simulink model "pipline_system"  (R2022b)
settings: Solver=FixedStepAuto  StartTime=0.0  StopTime=2000  FixedStep=Ts  RelTol=1e-5
values from neighbouring files (symbols this model uses):
  Aeq = [A_bar -B_bar ... (first row only)    [run_pipeline_system.m]
  B = -[1;0;0;0]    [myStateTransitionFcn.m]    (also in run_pipeline_system.m = [1;0;0;0])
  B_dem = -[0;0;0;1]    [myStateTransitionFcn.m]    (also in run_pipeline_system.m = [0;0;0;1])
  B_dem_bar = kron(eye(h),B_demd)    [run_pipeline_system.m]
  B_h = -[0 0;1 0;0 1;0 0]    [myStateTransitionFcn.m]    (also in run_pipeline_system.m = [0 0;1 0;0 1;0 0])
  Bh_bar = kron(eye(h),B_hd)    [run_pipeline_system.m]
  c = 330    [myStateTransitionFcn.m]    (also in run_pipeline_system.m)
  h = 10    [run_pipeline_system.m]
  K_control = place(A,B,poles)    [run_pipeline_system.m]
  K_inv = (pi^2)/(64*c^2)*f*D_edge.^5./L_edge    [myStateTransitionFcn.m]    (also in run_pipeline_system.m)
  M = blkdiag(Q_bar, R_bar)    [run_pipeline_system.m]
  n = 4    [run_pipeline_system.m]
  p_eq = [P1;P2;P3;P4]    [run_pipeline_system.m]
  V = (pi/8)*sum(((D_edge.^2).*L_edge),2,'omitnan')    [myStateTransitionFcn.m]    (also in run_pipeline_system.m)
  w_eq = c^2*(sqrt(K_inv.*abs(l*(p_eq.^2).' - (p_eq.^2)*l.')).*sign(l*p_eq.' - p_eq*l.')*l)./V    [run_pipeline_system.m]
undefined symbols (not defined in the file or in its folder): sigbuilder_block
settings Model: Creator=Anubi  LastModifiedBy=digitalstorm
settings ModelReferenceCC: EnableRefExpFcnMdlSchedulingChecks=on

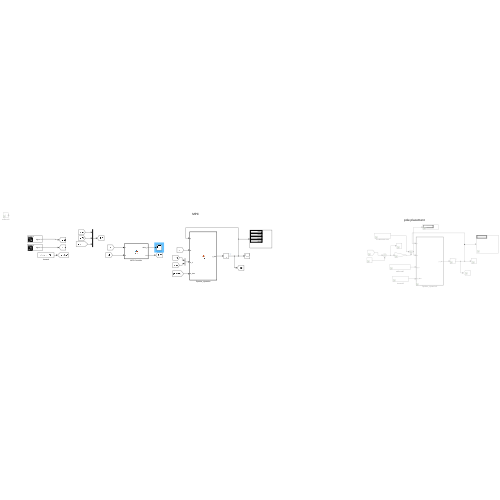
[thumbnail: Simulink's stored preview of the top-level diagram]
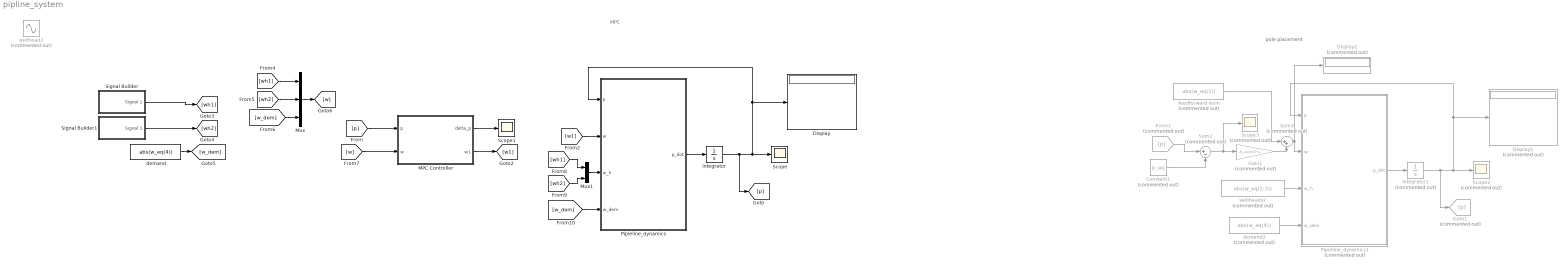
== system pipline_system ==
  note: pole placement
  note: MPC
  Constant1 : Constant  Commented=on  Value=p_eq
  Display : Display
  Display1 : Display  Commented=on
  Display2 : Display  Commented=on
  From1 : From  Commented=on  GotoTag=p
  Gain1 : Gain  Commented=on  Gain=-K_control  Multiplication=Matrix(K*u) (u vector)
  Goto1 : Goto  Commented=on  GotoTag=p
  Integrator : Integrator  InitialCondition=p_eq
  Integrator1 : Integrator  Commented=on  InitialCondition=0.5*p_eq
  MPC Controller : MATLAB Function  TreatAsAtomicUnit=on
  Mux : Mux  Inputs=3
  Mux1 : Mux  Inputs=2
  Pipieline_dynamics : MATLAB Function  TreatAsAtomicUnit=on
  Pipieline_dynamics1 : MATLAB Function  Commented=on  TreatAsAtomicUnit=on
  Scope : Scope
  Scope1 : Scope
  Scope2 : Scope  Commented=on
  Scope3 : Scope  Commented=on
  Signal Builder : Subsystem  Tag=STV Subsys  LoadFcn=sigbuilder_block('load');  StartFcn=sigbuilder_block('start');  StopFcn=sigbuilder_block('stop');  ClipboardFcn=sigbuilder_block('clipboard');  mask(Sigbuilder block){tuvar=[0:10]}
      mask help: Simulink:masks:SigbuilderBlock_MD
      mask init:
      | if ~strcmp(get_param(bdroot(gcbh),'SimulationStatus'),'stopped') tuvar = sigbuilder_block('maskInit'); end
      settings: CopyFcn=sigbuilder_block('copy');  DeleteFcn=sigbuilder_block('delete');  ModelCloseFcn=sigbuilder_block('modelClose');  PreSaveFcn=sigbuilder_block('preSave');  PauseFcn=sigbuilder_block('pause');  ContinueFcn=sigbuilder_block('continue');  NameChangeFcn=sigbuilder_block('namechange');  OpenFcn=sigbuilder_block('open',[428.444 190.222 568.889 387.556 ]);  CloseFcn=sigbuilder_block('close');
      mask Display: plot(0, 0, 100, 100,[2, 2, 32, 32, 2], [68, 8, 8, 68, 68],[32, 2], [38, 38], [32, 19, 2],[53, 60, 44], [32, 17, 17, 2],[16, 16, 31, 31]);txt = getActiveGroup(gcbh);text(2, 100, txt,'verticalAlignment', 'top');
  Signal Builder1 : Subsystem  Tag=STV Subsys  LoadFcn=sigbuilder_block('load');  StartFcn=sigbuilder_block('start');  StopFcn=sigbuilder_block('stop');  ClipboardFcn=sigbuilder_block('clipboard');  mask(Sigbuilder block){tuvar=[0:10]}
      mask help: Simulink:masks:SigbuilderBlock_MD
      mask init:
      | if ~strcmp(get_param(bdroot(gcbh),'SimulationStatus'),'stopped') tuvar = sigbuilder_block('maskInit'); end
      settings: CopyFcn=sigbuilder_block('copy');  DeleteFcn=sigbuilder_block('delete');  ModelCloseFcn=sigbuilder_block('modelClose');  PreSaveFcn=sigbuilder_block('preSave');  PauseFcn=sigbuilder_block('pause');  ContinueFcn=sigbuilder_block('continue');  NameChangeFcn=sigbuilder_block('namechange');  OpenFcn=sigbuilder_block('open',[428.444 190.222 568.889 387.556 ]);  CloseFcn=sigbuilder_block('close');
      mask Display: plot(0, 0, 100, 100,[2, 2, 32, 32, 2], [68, 8, 8, 68, 68],[32, 2], [38, 38], [32, 19, 2],[53, 60, 44], [32, 17, 17, 2],[16, 16, 31, 31]);txt = getActiveGroup(gcbh);text(2, 100, txt,'verticalAlignment', 'top');
  Sum2 : Sum  Commented=on  Inputs=|+-
  Sum3 : Sum  Commented=on  Inputs=|++
  demand : Constant  Value=abs(w_eq(4))
  demand2 : Constant  Commented=on  Value=abs(w_eq(4))
  feedforward term : Constant  Commented=on  Value=abs(w_eq(1))
  wellhead2 : Sin  Commented=on  Amplitude=2.5  Bias=5  Frequency=0.005  SampleTime=0
  wellheads2 : Constant  Commented=on  Value=abs(w_eq(2:3))
  wires:
  Pipieline_dynamics/1(p_dot) -> Integrator/1
  Integrator/1 -> [p], Scope/1, Pipieline_dynamics/1(p), Display/1
  Sum3/1 -> Display2/1, Pipieline_dynamics1/2(w)
  Gain1/1 -> Sum3/2
  feedforward term/1 -> Sum3/1
  demand2/1 -> Pipieline_dynamics1/4(w_dem)
  Sum2/1 -> Scope3/1, Gain1/1
  Integrator1/1 -> Goto1/1, Scope2/1, Pipieline_dynamics1/1(p), Display1/1
  wellheads2/1 -> Pipieline_dynamics1/3(w_h)
  Pipieline_dynamics1/1(p_dot) -> Integrator1/1
  From1/1 -> Sum2/1
  Constant1/1 -> Sum2/2
  [p] -> MPC Controller/1(p)
  MPC Controller/2(w1) -> [w1]
  [w1] -> Pipieline_dynamics/2(w)
  demand/1 -> [w_dem]
  Mux/1 -> [w]
  [w] -> MPC Controller/2(w)
  Mux1/1 -> Pipieline_dynamics/3(w_h)
  [wh1] -> Mux1/1
  [wh2] -> Mux1/2
  [w_dem] -> Pipieline_dynamics/4(w_dem)
  [wh1] -> Mux/1
  [wh2] -> Mux/2
  [w_dem] -> Mux/3
  MPC Controller/1(delta_p) -> Scope1/1
  Signal Builder/1(Signal 1) -> [wh1]
  Signal Builder1/1(Signal 1) -> [wh2]

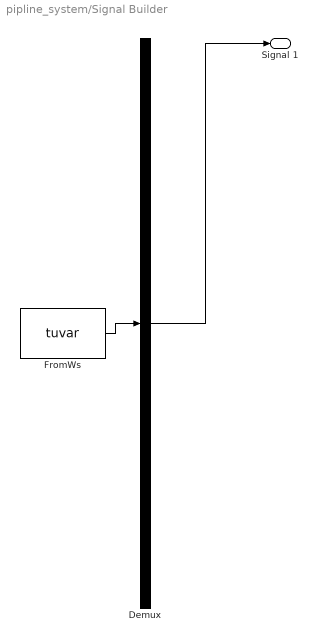
== system pipline_system/Signal Builder ==
  Demux : Demux  Tag=STV Demux  Outputs=1
      settings: DisplayOption=none
  FromWs : FromWorkspace  Tag=STV FromWs  VariableName=tuvar
      SigBuilderData=|
      | common.afterFinalStr = 'Extrapolate'
      | common.sampleTime = 0
      | dataSet.timeRange = [0 2000]
      | dataSet.name = 'Group 1'
      | sbobj.Groups.Name = 'Group 1'
      | sbobj.Groups.Signals.Name = 'Signal 1'
      | sbobj.Groups.Signals.XData = [0 1000 2000]
      | sbobj.Groups.Signals.YData = [5 4.8 5.1]
      | sbobj.Groups.TimeRange = [0 2000]
  Signal 1 : Outport  Tag=STV Outport
  wires:
  Demux/1 -> Signal 1/1
  FromWs/1 -> Demux/1

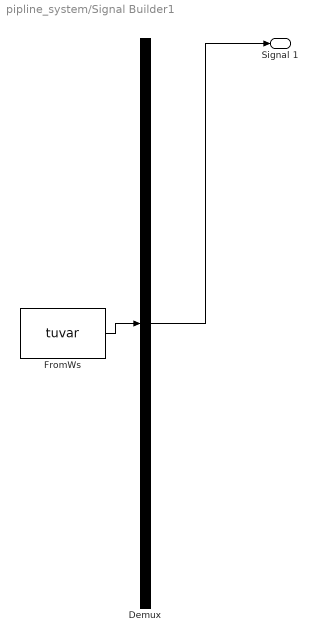
== system pipline_system/Signal Builder1 ==
  Demux : Demux  Tag=STV Demux  Outputs=1
      settings: DisplayOption=none
  FromWs : FromWorkspace  Tag=STV FromWs  VariableName=tuvar
      SigBuilderData=|
      | common.afterFinalStr = 'Extrapolate'
      | common.sampleTime = 0
      | dataSet.timeRange = [0 2000]
      | dataSet.name = 'Group 1'
      | sbobj.Groups.Name = 'Group 1'
      | sbobj.Groups.Signals.Name = 'Signal 1'
      | sbobj.Groups.Signals.XData = [0 1000 2000]
      | sbobj.Groups.Signals.YData = [5 4.8 5.1]
      | sbobj.Groups.TimeRange = [0 2000]
  Signal 1 : Outport  Tag=STV Outport
  wires:
  Demux/1 -> Signal 1/1
  FromWs/1 -> Demux/1

== matlab function pipline_system/Pipieline_dynamics1 ==
  data: p input; p_dot output; w input; w_h input; w_dem input; K_inv parameter; c parameter; V parameter; B_h parameter; B_dem parameter; B parameter
function p_dot = fcn(p,w,w_h,w_dem,K_inv, c, V, B_h, B_dem, B)
% COMMENTS HERE

p_sq = p.^2;
l    = ones(length(p),1);  % vector of ones
Psi = sqrt(K_inv.*abs(l*p_sq.' - p_sq*l.')).*sign(l*p.' - p*l.');

p_dot = c^2*(Psi*l)./V + B_h*w_h - B_dem*w_dem + B*w;

== matlab function pipline_system/Pipieline_dynamics ==
  data: p input; p_dot output; w input; w_h input; w_dem input; K_inv parameter; c parameter; V parameter; B_h parameter; B_dem parameter; B parameter
function p_dot = fcn(p,w,w_h,w_dem,K_inv, c, V, B_h, B_dem, B)
% COMMENTS HERE

p_sq = p.^2;
l    = ones(length(p),1);  % vector of ones
Psi = sqrt(K_inv.*abs(l*p_sq.' - p_sq*l.')).*sign(l*p.' - p*l.');

p_dot = c^2*(Psi*l)./V + B_h*w_h - B_dem*w_dem + B*w;

== matlab function pipline_system/MPC Controller ==
  data: delta_p output; p input; w input; w1 output; p_eq parameter; w_eq parameter; M parameter; Aeq parameter; Bh_bar parameter; B_dem_bar parameter; n parameter; h parameter
function [delta_p,w1] = fcn(p,w,p_eq, w_eq, M, Aeq, Bh_bar, B_dem_bar, n, h)

coder.extrinsic('MPC_control');

%% formulate rest MPC parameters
delta_p = p-p_eq;
delta_w = w-abs(w_eq(2:end));
beq1 = [Bh_bar -B_dem_bar]*kron(ones(h,1),delta_w);
beq2 = -delta_p;
beq = [beq1;beq2];

%% call solver
z = zeros(size(M,1),1);   % z = [delta_p; delta_w]
z(:) = MPC_control(M,Aeq,beq);
delta_w1 = z(n*h+1);


%% add feedfowward term
w1 = delta_w1 + abs(w_eq(1));
